simulink model "RRpendulum_sine_input"  (R2024b)
settings: Solver=VariableStepAuto  StartTime=0.0  StopTime=15  RelTol=1e-7  AbsTol=1e-8
undefined symbols (not defined in the file): b1_num, b2_num, g_num, m_num, q1_0, q2_0, v1_0, v1ampl, v1freq, v2_0
libraries: digtwin_labo_lib x1
settings Model: Creator=u0130154  LastModifiedBy=u0130154
settings SimscapeCC: SimscapeLogType=all

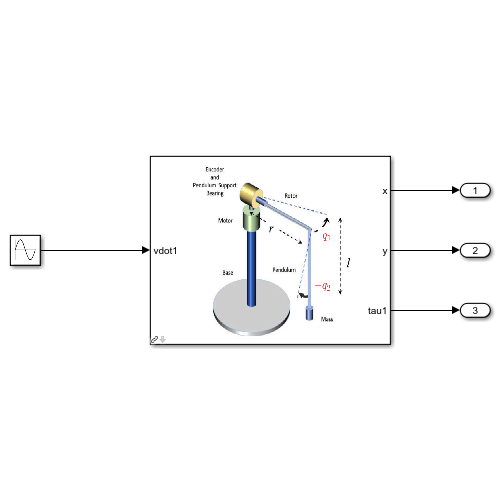
[thumbnail: Simulink's stored preview of the top-level diagram]
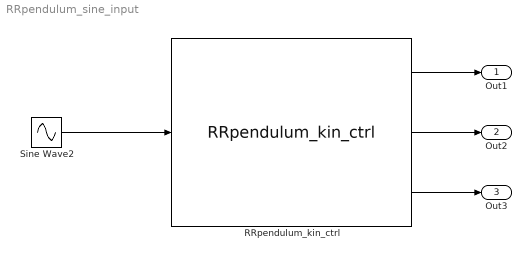
== system RRpendulum_sine_input ==
  RRpendulum_kin_ctrl : digtwin_labo_lib/RRpendulum_kin_ctrl  initstate=[q1_0; v1_0 ;q2_0; v2_0]  satlimits=satlimits  g=g_num  m=m_num  r=r_num  l=l_num  b=[b1_num b2_num]
  Sine Wave2 : Sin  Amplitude=v1ampl*2*pi*v1freq  Frequency=2*pi*v1freq  Phase=pi/2  SampleTime=0
  Out1 : Outport
  Out2 : Outport  Port=2
  Out3 : Outport  Port=3
  wires:
  RRpendulum_kin_ctrl/2 -> Out2/1
  RRpendulum_kin_ctrl/1 -> Out1/1
  RRpendulum_kin_ctrl/3 -> Out3/1
  Sine Wave2/1 -> RRpendulum_kin_ctrl/1
